simulink model "qiita1"  (R2019a)
settings: Solver=FixedStepDiscrete  StartTime=0.0  StopTime=Inf  FixedStep=0.01  RelTol=1e-3  EnableMultiTasking=on
libraries: mcp2515lib x11, simulink x8, svdutilitieslib x1, robotlib x1
settings Model: Creator=tatsuyai  LastModifiedBy=tatsuyai
settings SolverCC: PositivePriorityOrder=on
settings OptimizationCC: EnhancedBackFolding=on  PassReuseOutputArgsAs=Individual arguments  MaxStackSize=64  OptimizeBlockOrder=speed  DifferentSizesBufferReuse=on  OptimizationCustomize=off
settings DebuggingCC: ParameterTunabilityLossMsg=error
settings HardwareCC: ProdBitPerPointer=32  ProdBitPerSizeT=32  ProdBitPerPtrDiffT=32  ProdLargestAtomicInteger=Long  ProdLargestAtomicFloat=Double  ProdWordSize=32  ProdHWDeviceType=ARM Compatible->ARM Cortex  UseEmbeddedCoderFeatures=off  UseSimulinkCoderFeatures=off
settings SFSimCC: MATLABDynamicMemAlloc=off
settings RTWCC: SystemTargetFile=ert.tlc  HardwareBoard=Raspberry Pi - Robot Operating System (ROS)  TLCOptions="-aInlineSetEventsForThisBaseRateFcn=TLC_FALSE -aSuppressMultiTaskScheduler=TLC_FALSE  -aRateBasedStepFcn=0"  TemplateMakefile=ert_default_tmf  GenerateReport=on  Toolchain=Catkin  IncludeHyperlinkInReport=on  LaunchReport=on  TargetLang=C++  GenerateTraceInfo=on  GenerateTraceReport=on  GenerateTraceReportSl=on  GenerateTraceReportSf=on  GenerateTraceReportEml=on
settings CodeAppCC: ForceParamTrailComments=on  IgnoreCustomStorageClasses=off  OperatorAnnotations=on  SimulinkDataObjDesc=on  SFDataObjDesc=on  InsertBlockDesc=on
settings ERTTargetCC: SupportNonInlinedSFcns=on

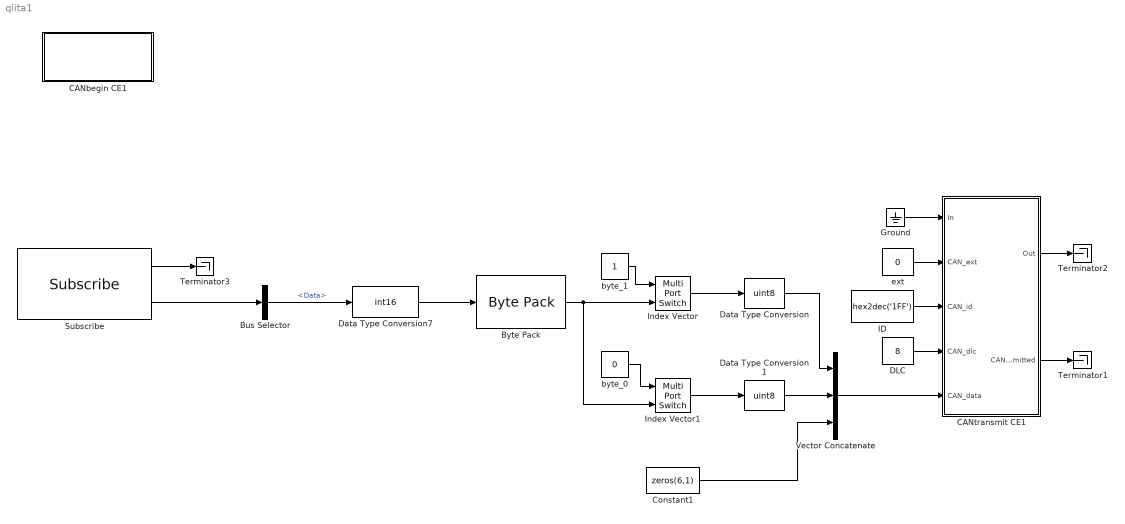
== system qiita1 ==
  Bus Selector : BusSelector  OutputSignals=Data
  Byte Pack : svdutilitieslib/Byte Pack  maskPackedDataType=uint8  datatypes={'int16'}  byteAlign=1  blockPlatform=arduinoert
      settings: SourceProductName=Embedded Coder Support Package for ARM Cortex-A Processors  SourceProductBaseCode=ECCORTEXA
  CANbegin CE1 : Subsystem  TreatAsAtomicUnit=on  mask{TargetHardware=Raspberry Pi, Oscillator=16, CANSpeed=1000, CSpin=10}
      mask prompts: TargetHardware "Target Hardware"; Oscillator "Oscillator frequency(MHz)"; CANSpeed "CAN speed(kHz)"; CSpin "Chip Select Pin"
      mask init:
      | % Get this mask's handle
      | maskObj = Simulink.Mask.get(gcb);
      | 
      | % Get the selected value from mask parameter's option
      | str_TargetHard = char(maskObj.Parameters(1).TypeOptions(TargetHardware));
      | str_Osc = char(maskObj.Parameters(2).TypeOptions(Oscillator));
      | str_CANSpeed = char(maskObj.Parameters(3).TypeOptions(CANSpeed));
      | 
      | % Set Icon
      | str1 = sprintf('%s(Model)',str_TargetHard);
      | str2 = sprintf('Oscillator: %s(MHz)',str_Osc);
      | str3 = sprintf('CAN Bus Speed: %s(kHz)',str_CANSpeed);
      | str4 = sprintf('Chip Select pin: %d',CSpin);
      | 
      | % Set the values of Variant Subsystem
      | switch str_TargetHard
      |     case 'Arduino'
      |         str = [str1,'\n',str2,'\n',str3,'\n',str4];
      |         evalin('base',sprintf('CSpin = %d;',CSpin));        
      |         evalin('base','Hardware = 1;');
      |     case 'Raspberry Pi'
      |         str = [str1,'\n',str2,'\n',str3];
      |         evalin('base',sprintf('clear CSpin',CSpin));           
      |         evalin('base','Hardware = 2;');     
      | end  
      | 
      | % Get the CAN Configuration register's value from mask parameter's option
      | if str_Osc == '8' %[MHz]
      |     switch str_CANSpeed
      |         case '1000'
      |             BPR = 0; PHSEG1 = 0; PRSEG = 0; PHSEG2 = 0;
      |         case '500'
      |             BPR = 0; PHSEG1 = 2; PRSEG = 0; PHSEG2 = 2;
      |         case '250'
      |             BPR = 0; PHSEG1 = 6; PRSEG = 0; PHSEG2 = 6;
      |         case '125'
      |             BPR = 1; PHSEG1 = 6; PRSEG = 1; PHSEG2 = 5;
      |         case '100'
      |             BPR = 1; PHSEG1 = 7; PRSEG = 2; PHSEG2 = 7;
      |         case '83.3'
      |             BPR = 1; PHSEG1 = 7; PRSEG = 6; PHSEG2 = 7;
      |         case '62.5'
      |             BPR = 3; PHSEG1 = 6; PRSEG = 0; PHSEG2 = 6;
      |         case '50'
      |             BPR = 3; PHSEG1 = 7; PRSEG = 2; PHSEG2 = 7;
      |         case '33.3'
      |             BPR = 4; PHSEG1 = 7; PRSEG = 6; PHSEG2 = 7;
      |     end            
      | elseif str_Osc == '16' %[MHz]
      |     switch str_CANSpeed  
      |         case '1000'
      |             BPR = 0; PHSEG1 = 2; PRSEG = 0; PHSEG2 = 2;
      |         case '500'
      |             BPR = 0; PHSEG1 = 6; PRSEG = 0; PHSEG2 = 6;
      |         case '250'
      |             BPR = 1; PHSEG1 = 6; PRSEG = 1; PHSEG2 = 5;        
      |         case '125'
      |             BPR = 3; PHSEG1 = 6; PRSEG = 0; PHSEG2 = 6;
      |         case '100'
      |             BPR = 3; PHSEG1 = 7; PRSEG = 2; PHSEG2 = 7;
      |         case '83.3'
      |             BPR = 3; PHSEG1 = 7; PRSEG = 6; PHSEG2 = 7;
      |         case '62.5'
      |             BPR = 7; PHSEG1 = 6; PRSEG = 0; PHSEG2 = 6;
      |         case '50'
      |             BPR = 7; PHSEG1 = 7; PRSEG = 2; PHSEG2 = 7;
      |         case '33.3'
      |             BPR = 9; PHSEG1 = 7; PRSEG = 6; PHSEG2 = 7;        
      |     end   
      | end
      | % Set the CAN Configuration register's value
      | address2A = BPR;          % bit7-6 :SJW, bit5-0: BPR
      | address29 = 192 ...       % bit7: BTLMODE = 1, bit6:SAM = 1
      |             + 8*PHSEG1 ...% bit5-3: PHSEG1
      |             +PRSEG;       % bit2-0: PRSEG
      | address28 = 128 ...       % bit7: SOF = 1, bit6:WAKFIL = 0
      |             + PHSEG2;     % bit5-3: 0, bit2-0: PHSEG2
      settings: RTWSystemCode=Nonreusable function
      mask TypeOptions TargetHardware: Arduino | Raspberry Pi
      mask Callback TargetHardware:
      | if(strcmp(get_param(gcb,'TargetHardware'),'Arduino'))
      |     set_param(gcb,'MaskVisibilities',{'on','on','on','on'})
      | else
      |     set_param(gcb,'MaskVisibilities',{'on','on','on','off'})
      | end
      mask TypeOptions Oscillator: 8 | 16
      mask TypeOptions CANSpeed: 1000 | 500 | 250 | 125 | 100 | 83.3 | 62.5 | 50 | 33.3
      mask DialogControl DescGroupVar Prompt: Description
      mask DialogControl DescTextVar Prompt: This block must be executed only once when beginning CAN communication because MCP2515’s register needs to be configured. And the frequency of oscillator for MCP2515 is also needed because it effects to the setting parameters of MCP2515's register.
      mask Display: disp(str)
  CANtransmit CE1 : Subsystem  TreatAsAtomicUnit=on
      mask DialogControl DescGroupVar Prompt: Description
      mask DialogControl DescTextVar Prompt: CANtransmit inputs CAN data by converting MCP2515 TX buffer register’s values. In/Out ports are no use because they are used for controlling the execution order. CAN_Transmitted outputs 1(Success) or 2(Fail).
  Constant1 : Constant  Value=zeros(6,1)  OutDataTypeStr=uint8
  DLC : Constant  Value=8  OutDataTypeStr=uint8
  Data Type Conversion : DataTypeConversion  OutDataTypeStr=uint8
  Data Type Conversion1 : DataTypeConversion  OutDataTypeStr=uint8
  Data Type Conversion7 : DataTypeConversion  OutDataTypeStr=int16
  Ground : Ground
  ID : Constant  Value=hex2dec('1FF')  OutDataTypeStr=uint32
  Index Vector : MultiPortSwitch  DataPortOrder=Zero-based contiguous  Inputs=1  zeroidx=on
  Index Vector1 : MultiPortSwitch  DataPortOrder=Zero-based contiguous  Inputs=1  zeroidx=on
  Subscribe : robotlib/Subscribe  topicSource=Specify your own  topic=/gm6020_1/cmd_voltage  messageType=std_msgs/Int16  sampleTime=-1  messageQueueLength=1
      settings: SourceProductName=ROS Toolbox
  Terminator1 : Terminator
  Terminator2 : Terminator
  Terminator3 : Terminator
  Vector Concatenate : Concatenate  NumInputs=3
  byte_0 : Constant  Value=0  OutDataTypeStr=uint8
  byte_1 : Constant  OutDataTypeStr=uint8
  ext : Constant  Value=0  OutDataTypeStr=uint8
  wires:
  Ground/1 -> CANtransmit CE1/1(In)
  Vector Concatenate/1 -> CANtransmit CE1/5(CAN_data)
  ext/1 -> CANtransmit CE1/2(CAN_ext)
  Data Type Conversion7/1 -> Byte Pack/1
  byte_0/1 -> Index Vector1/1
  Index Vector/1 -> Data Type Conversion/1
  Data Type Conversion1/1 -> Vector Concatenate/2
  Constant1/1 -> Vector Concatenate/3
  Data Type Conversion/1 -> Vector Concatenate/1
  CANtransmit CE1/2(CAN_Transmitted) -> Terminator1/1
  ID/1 -> CANtransmit CE1/3(CAN_id)
  byte_1/1 -> Index Vector/1
  CANtransmit CE1/1(Out) -> Terminator2/1
  DLC/1 -> CANtransmit CE1/4(CAN_dlc)
  Index Vector1/1 -> Data Type Conversion1/1
  Byte Pack/1 -> Index Vector1/2, Index Vector/2
  Subscribe/2 -> Bus Selector/1
  Bus Selector/1 -> Data Type Conversion7/1  "<Data>"
  Subscribe/1 -> Terminator3/1

== system qiita1/CANbegin CE1 ==
  Constant : Constant  Value=0  OutDataTypeStr=boolean  SampleTime=-1
  Temporary buffer : DataStoreMemory  DataStoreName=temp_1byte  ReadBeforeWriteMsg=warning  WriteAfterWriteMsg=warning  WriteAfterReadMsg=warning  ShowAdditionalParam=off  OutDataTypeStr=uint8
  Unit Delay : UnitDelay  InitialCondition=1  SampleTime=-1  HasFrameUpgradeWarning=on
  setup : Subsystem  TreatAsAtomicUnit=on
      settings: RTWSystemCode=Nonreusable function  RTWFileNameOpts=Use subsystem name
  wires:
  Unit Delay/1 -> setup/Enable
  Constant/1 -> Unit Delay/1

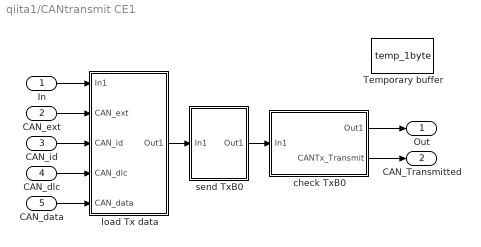
== system qiita1/CANtransmit CE1 ==
  In : Inport
  CAN_ext : Inport  Port=2
  CAN_id : Inport  Port=3
  CAN_dlc : Inport  Port=4
  CAN_data : Inport  Port=5
  Temporary buffer : DataStoreMemory  DataStoreName=temp_1byte  ReadBeforeWriteMsg=warning  WriteAfterWriteMsg=warning  WriteAfterReadMsg=warning  ShowAdditionalParam=off  OutDataTypeStr=uint8
  check TxB0 : Subsystem  TreatAsAtomicUnit=on
  load Tx data : Subsystem  TreatAsAtomicUnit=on
  send TxB0 : Subsystem  TreatAsAtomicUnit=on
  Out : Outport
  CAN_Transmitted : Outport  Port=2
  wires:
  In/1 -> load Tx data/1(In1)
  load Tx data/1(Out1) -> send TxB0/1(In1)
  send TxB0/1(Out1) -> check TxB0/1(In1)
  check TxB0/1(Out1) -> Out/1
  check TxB0/2(CANTx_Transmit) -> CAN_Transmitted/1
  CAN_ext/1 -> load Tx data/2(CAN_ext)
  CAN_id/1 -> load Tx data/3(CAN_id)
  CAN_dlc/1 -> load Tx data/4(CAN_dlc)
  CAN_data/1 -> load Tx data/5(CAN_data)

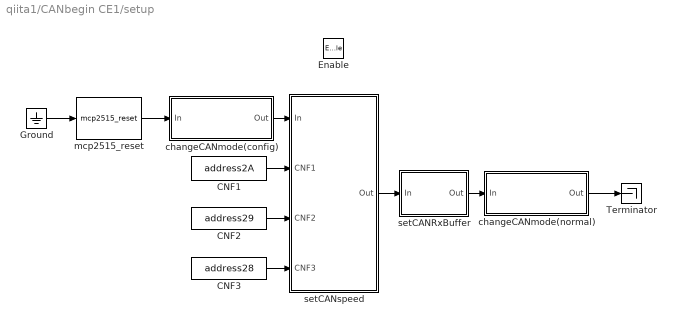
== system qiita1/CANbegin CE1/setup ==
  Enable : EnablePort
  CNF1 : Constant  Value=address2A  OutDataTypeStr=uint8
  CNF2 : Constant  Value=address29  OutDataTypeStr=uint8
  CNF3 : Constant  Value=address28  OutDataTypeStr=uint8
  Ground : Ground
  Terminator : Terminator
  changeCANmode(config) : Subsystem  TreatAsAtomicUnit=on
  changeCANmode(normal) : Subsystem  TreatAsAtomicUnit=on
  mcp2515_reset : mcp2515lib/CAN application/mcp2515 driver CE1/mcp2515_reset  SystemSampleTime=-1
      settings: SourceProductName=CAN device driver for mcp2515
  setCANRxBuffer : Subsystem  TreatAsAtomicUnit=on
  setCANspeed : Subsystem  TreatAsAtomicUnit=on
  wires:
  CNF3/1 -> setCANspeed/4(CNF3)
  CNF2/1 -> setCANspeed/3(CNF2)
  CNF1/1 -> setCANspeed/2(CNF1)
  mcp2515_reset/1 -> changeCANmode(config)/1(In)
  changeCANmode(config)/1(Out) -> setCANspeed/1(In)
  setCANspeed/1(Out) -> setCANRxBuffer/1(In)
  setCANRxBuffer/1(Out) -> changeCANmode(normal)/1(In)
  Ground/1 -> mcp2515_reset/1
  changeCANmode(normal)/1(Out) -> Terminator/1

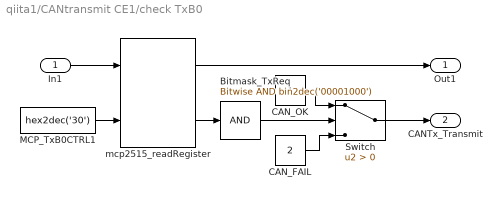
== system qiita1/CANtransmit CE1/check TxB0 ==
  In1 : Inport
  Bitmask_TxReq : simulink/Logic and Bit Operations/Bitwise Operator  logicop=AND  UseBitMask=on  BitMask=bin2dec('00001000')  BitMaskRealWorld=Stored Integer
  CAN_FAIL : Constant  Value=2  OutDataTypeStr=int8
  CAN_OK : Constant  OutDataTypeStr=int8
  MCP_TxB0CTRL1 : Constant  Value=hex2dec('30')  OutDataTypeStr=uint8
  Switch : Switch  Criteria=u2 > Threshold
  mcp2515_readRegister : mcp2515lib/CAN application/mcp2515 driver CE1/mcp2515_readRegister  SystemSampleTime=-1
      settings: SourceProductName=CAN device driver for mcp2515
  Out1 : Outport
  CANTx_Transmit : Outport  Port=2
  wires:
  CAN_FAIL/1 -> Switch/3
  mcp2515_readRegister/1 -> Out1/1
  mcp2515_readRegister/2 -> Bitmask_TxReq/1
  MCP_TxB0CTRL1/1 -> mcp2515_readRegister/2
  Bitmask_TxReq/1 -> Switch/2
  Switch/1 -> CANTx_Transmit/1
  CAN_OK/1 -> Switch/1
  In1/1 -> mcp2515_readRegister/1

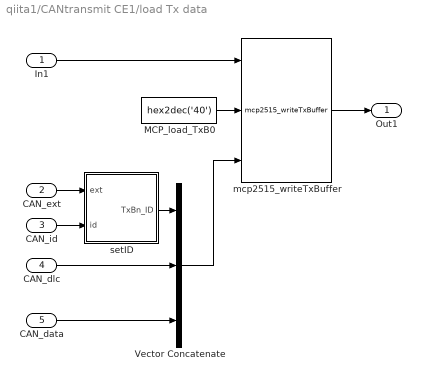
== system qiita1/CANtransmit CE1/load Tx data ==
  In1 : Inport
  CAN_ext : Inport  Port=2
  CAN_id : Inport  Port=3
  CAN_dlc : Inport  Port=4
  CAN_data : Inport  Port=5
  MCP_load_TxB0 : Constant  Value=hex2dec('40')  OutDataTypeStr=uint8
  Vector Concatenate : Concatenate  NumInputs=3
  mcp2515_writeTxBuffer : mcp2515lib/CAN application/mcp2515 driver CE1/mcp2515_writeTxBuffer  SystemSampleTime=-1
      settings: SourceProductName=CAN device driver for mcp2515
  setID : Subsystem  TreatAsAtomicUnit=on
      settings: RTWSystemCode=Inline
  Out1 : Outport
  wires:
  CAN_ext/1 -> setID/1(ext)
  CAN_id/1 -> setID/2(id)
  CAN_data/1 -> Vector Concatenate/3
  CAN_dlc/1 -> Vector Concatenate/2
  setID/1(TxBn_ID) -> Vector Concatenate/1
  In1/1 -> mcp2515_writeTxBuffer/1
  mcp2515_writeTxBuffer/1 -> Out1/1
  MCP_load_TxB0/1 -> mcp2515_writeTxBuffer/2
  Vector Concatenate/1 -> mcp2515_writeTxBuffer/3

== system qiita1/CANtransmit CE1/send TxB0 ==
  In1 : Inport
  MCP_TxB0CTRL : Constant  Value=hex2dec('30')  OutDataTypeStr=uint8
  TxREQ : Constant  Value=8  OutDataTypeStr=uint8
  mcp2515_writeRegister1 : mcp2515lib/CAN application/mcp2515 driver CE1/mcp2515_writeRegister  SystemSampleTime=-1
      settings: SourceProductName=CAN device driver for mcp2515
  Out1 : Outport
  wires:
  MCP_TxB0CTRL/1 -> mcp2515_writeRegister1/2
  mcp2515_writeRegister1/1 -> Out1/1
  In1/1 -> mcp2515_writeRegister1/1
  TxREQ/1 -> mcp2515_writeRegister1/3

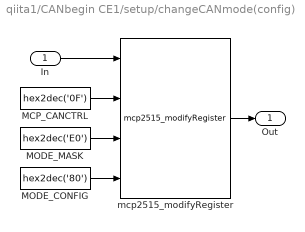
== system qiita1/CANbegin CE1/setup/changeCANmode(config) ==
  In : Inport
  MCP_CANCTRL : Constant  Value=hex2dec('0F')  OutDataTypeStr=uint8
  MODE_CONFIG : Constant  Value=hex2dec('80')  OutDataTypeStr=uint8
  MODE_MASK : Constant  Value=hex2dec('E0')  OutDataTypeStr=uint8
  mcp2515_modifyRegister : mcp2515lib/CAN application/mcp2515 driver CE1/mcp2515_modifyRegister  SystemSampleTime=-1
      settings: SourceProductName=CAN device driver for mcp2515
  Out : Outport
  wires:
  MODE_CONFIG/1 -> mcp2515_modifyRegister/4
  MODE_MASK/1 -> mcp2515_modifyRegister/3
  MCP_CANCTRL/1 -> mcp2515_modifyRegister/2
  In/1 -> mcp2515_modifyRegister/1
  mcp2515_modifyRegister/1 -> Out/1

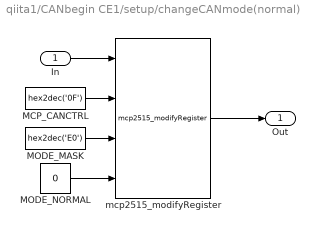
== system qiita1/CANbegin CE1/setup/changeCANmode(normal) ==
  In : Inport
  MCP_CANCTRL : Constant  Value=hex2dec('0F')  OutDataTypeStr=uint8
  MODE_MASK : Constant  Value=hex2dec('E0')  OutDataTypeStr=uint8
  MODE_NORMAL : Constant  Value=0  OutDataTypeStr=uint8
  mcp2515_modifyRegister : mcp2515lib/CAN application/mcp2515 driver CE1/mcp2515_modifyRegister  SystemSampleTime=-1
      settings: SourceProductName=CAN device driver for mcp2515
  Out : Outport
  wires:
  MODE_MASK/1 -> mcp2515_modifyRegister/3
  MODE_NORMAL/1 -> mcp2515_modifyRegister/4
  MCP_CANCTRL/1 -> mcp2515_modifyRegister/2
  In/1 -> mcp2515_modifyRegister/1
  mcp2515_modifyRegister/1 -> Out/1

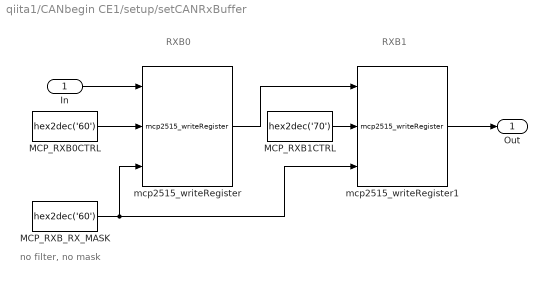
== system qiita1/CANbegin CE1/setup/setCANRxBuffer ==
  note: RXB0
  note: RXB1
  note: no filter, no mask
  In : Inport
  MCP_RXB0CTRL : Constant  Value=hex2dec('60')  OutDataTypeStr=uint8
  MCP_RXB1CTRL : Constant  Value=hex2dec('70')  OutDataTypeStr=uint8
  MCP_RXB_RX_MASK : Constant  Value=hex2dec('60')  OutDataTypeStr=uint8
  mcp2515_writeRegister : mcp2515lib/CAN application/mcp2515 driver CE1/mcp2515_writeRegister  SystemSampleTime=-1
      settings: SourceProductName=CAN device driver for mcp2515
  mcp2515_writeRegister1 : mcp2515lib/CAN application/mcp2515 driver CE1/mcp2515_writeRegister  SystemSampleTime=-1
      settings: SourceProductName=CAN device driver for mcp2515
  Out : Outport
  wires:
  MCP_RXB0CTRL/1 -> mcp2515_writeRegister/2
  MCP_RXB1CTRL/1 -> mcp2515_writeRegister1/2
  MCP_RXB_RX_MASK/1 -> mcp2515_writeRegister/3, mcp2515_writeRegister1/3
  In/1 -> mcp2515_writeRegister/1
  mcp2515_writeRegister1/1 -> Out/1
  mcp2515_writeRegister/1 -> mcp2515_writeRegister1/1

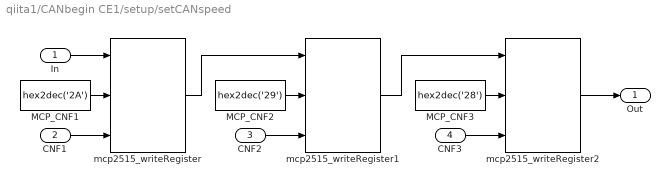
== system qiita1/CANbegin CE1/setup/setCANspeed ==
  In : Inport
  CNF1 : Inport  Port=2
  CNF2 : Inport  Port=3
  CNF3 : Inport  Port=4
  MCP_CNF1 : Constant  Value=hex2dec('2A')  OutDataTypeStr=uint8
  MCP_CNF2 : Constant  Value=hex2dec('29')  OutDataTypeStr=uint8
  MCP_CNF3 : Constant  Value=hex2dec('28')  OutDataTypeStr=uint8
  mcp2515_writeRegister : mcp2515lib/CAN application/mcp2515 driver CE1/mcp2515_writeRegister  SystemSampleTime=-1
      settings: SourceProductName=CAN device driver for mcp2515
  mcp2515_writeRegister1 : mcp2515lib/CAN application/mcp2515 driver CE1/mcp2515_writeRegister  SystemSampleTime=-1
      settings: SourceProductName=CAN device driver for mcp2515
  mcp2515_writeRegister2 : mcp2515lib/CAN application/mcp2515 driver CE1/mcp2515_writeRegister  SystemSampleTime=-1
      settings: SourceProductName=CAN device driver for mcp2515
  Out : Outport
  wires:
  MCP_CNF2/1 -> mcp2515_writeRegister1/2
  MCP_CNF3/1 -> mcp2515_writeRegister2/2
  CNF3/1 -> mcp2515_writeRegister2/3
  CNF1/1 -> mcp2515_writeRegister/3
  MCP_CNF1/1 -> mcp2515_writeRegister/2
  CNF2/1 -> mcp2515_writeRegister1/3
  In/1 -> mcp2515_writeRegister/1
  mcp2515_writeRegister/1 -> mcp2515_writeRegister1/1
  mcp2515_writeRegister1/1 -> mcp2515_writeRegister2/1
  mcp2515_writeRegister2/1 -> Out/1

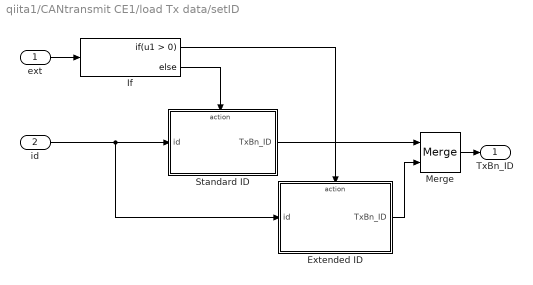
== system qiita1/CANtransmit CE1/load Tx data/setID ==
  ext : Inport
  id : Inport  Port=2
  Extended ID : Subsystem  TreatAsAtomicUnit=on
  If : If
  Merge : Merge
  Standard ID : Subsystem  TreatAsAtomicUnit=on
  TxBn_ID : Outport
  wires:
  ext/1 -> If/1
  If/1 -> Extended ID/Action
  If/2 -> Standard ID/Action
  Extended ID/1(TxBn_ID) -> Merge/2
  Standard ID/1(TxBn_ID) -> Merge/1
  Merge/1 -> TxBn_ID/1
  id/1 -> Extended ID/1(id), Standard ID/1(id)

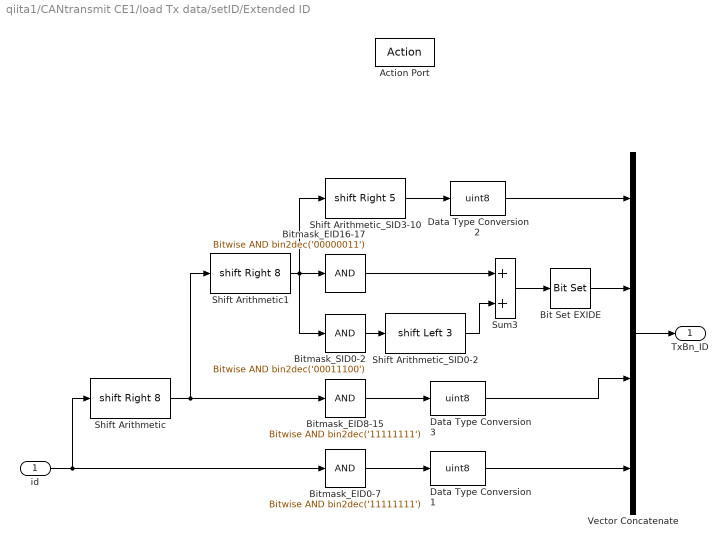
== system qiita1/CANtransmit CE1/load Tx data/setID/Extended ID ==
  id : Inport
  Action Port : ActionPort  ActionPortLabel=if(u1 > 0)
  Bit Set EXIDE : simulink/Logic and Bit Operations/Bit Set  iBit=3
      settings: SourceProductName=Simulink  SourceProductBaseCode=SL
  Bitmask_EID0-7 : simulink/Logic and Bit Operations/Bitwise Operator  logicop=AND  UseBitMask=on  BitMask=bin2dec('11111111')  BitMaskRealWorld=Stored Integer
  Bitmask_EID16-17 : simulink/Logic and Bit Operations/Bitwise Operator  logicop=AND  UseBitMask=on  BitMask=bin2dec('00000011')  BitMaskRealWorld=Stored Integer
  Bitmask_EID8-15 : simulink/Logic and Bit Operations/Bitwise Operator  logicop=AND  UseBitMask=on  BitMask=bin2dec('11111111')  BitMaskRealWorld=Stored Integer
  Bitmask_SID0-2 : simulink/Logic and Bit Operations/Bitwise Operator  logicop=AND  UseBitMask=on  BitMask=bin2dec('00011100')  BitMaskRealWorld=Stored Integer
  Data Type Conversion1 : DataTypeConversion  OutDataTypeStr=uint8  RndMeth=Simplest
  Data Type Conversion2 : DataTypeConversion  OutDataTypeStr=uint8  RndMeth=Simplest
  Data Type Conversion3 : DataTypeConversion  OutDataTypeStr=uint8  RndMeth=Simplest
  Shift Arithmetic : ArithShift  BitShiftNumber=8  BitShiftDirection=Right
  Shift Arithmetic1 : ArithShift  BitShiftNumber=8  BitShiftDirection=Right
  Shift Arithmetic_SID0-2 : ArithShift  BitShiftNumber=3  BitShiftDirection=Left
  Shift Arithmetic_SID3-10 : ArithShift  BitShiftNumber=5  BitShiftDirection=Right
  Sum3 : Sum  OutDataTypeStr=uint8
  Vector Concatenate : Concatenate  NumInputs=4
  TxBn_ID : Outport
  wires:
  Vector Concatenate/1 -> TxBn_ID/1
  id/1 -> Shift Arithmetic/1, Bitmask_EID0-7/1
  Bitmask_EID0-7/1 -> Data Type Conversion1/1
  Data Type Conversion1/1 -> Vector Concatenate/4
  Shift Arithmetic/1 -> Shift Arithmetic1/1, Bitmask_EID8-15/1
  Bitmask_EID8-15/1 -> Data Type Conversion3/1
  Data Type Conversion3/1 -> Vector Concatenate/3
  Shift Arithmetic1/1 -> Shift Arithmetic_SID3-10/1, Bitmask_SID0-2/1, Bitmask_EID16-17/1
  Sum3/1 -> Bit Set EXIDE/1
  Bitmask_EID16-17/1 -> Sum3/1
  Bitmask_SID0-2/1 -> Shift Arithmetic_SID0-2/1
  Shift Arithmetic_SID0-2/1 -> Sum3/2
  Bit Set EXIDE/1 -> Vector Concatenate/2
  Shift Arithmetic_SID3-10/1 -> Data Type Conversion2/1
  Data Type Conversion2/1 -> Vector Concatenate/1

== system qiita1/CANtransmit CE1/load Tx data/setID/Standard ID ==
  id : Inport
  Action Port : ActionPort  ActionPortLabel=else
  Vector Concatenate : Concatenate  NumInputs=4
  convert_ID : Subsystem  TreatAsAtomicUnit=on
  no data : Constant  Value=0  OutDataTypeStr=uint8
  TxBn_ID : Outport
  wires:
  Vector Concatenate/1 -> TxBn_ID/1
  no data/1 -> Vector Concatenate/3, Vector Concatenate/4
  convert_ID/2(SIDL) -> Vector Concatenate/2
  id/1 -> convert_ID/1(id)
  convert_ID/1(SIDH) -> Vector Concatenate/1

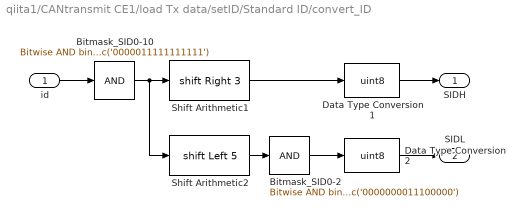
== system qiita1/CANtransmit CE1/load Tx data/setID/Standard ID/convert_ID ==
  id : Inport
  Bitmask_SID0-10 : simulink/Logic and Bit Operations/Bitwise Operator  logicop=AND  UseBitMask=on  BitMask=bin2dec('0000011111111111')  BitMaskRealWorld=Stored Integer
  Bitmask_SID0-2 : simulink/Logic and Bit Operations/Bitwise Operator  logicop=AND  UseBitMask=on  BitMask=bin2dec('0000000011100000')  BitMaskRealWorld=Stored Integer
  Data Type Conversion1 : DataTypeConversion  OutDataTypeStr=uint8  RndMeth=Simplest
  Data Type Conversion2 : DataTypeConversion  OutDataTypeStr=uint8  RndMeth=Simplest
  Shift Arithmetic1 : ArithShift  BitShiftNumber=3  BitShiftDirection=Right
  Shift Arithmetic2 : ArithShift  BitShiftNumber=5  BitShiftDirection=Left
  SIDH : Outport
  SIDL : Outport  Port=2
  wires:
  Shift Arithmetic1/1 -> Data Type Conversion1/1
  Data Type Conversion1/1 -> SIDH/1
  Bitmask_SID0-10/1 -> Shift Arithmetic2/1, Shift Arithmetic1/1
  Data Type Conversion2/1 -> SIDL/1
  Shift Arithmetic2/1 -> Bitmask_SID0-2/1
  id/1 -> Bitmask_SID0-10/1
  Bitmask_SID0-2/1 -> Data Type Conversion2/1
